simulink model "Force"  (R2016b)
settings: configuration reference "WheelSimConfiguration2016" (kept outside this file)
libraries: dspstat3 x1
settings Model: Creator=At  LastModifiedBy=ateay
settings ConfigSetRef: SourceLocation=Base Workspace

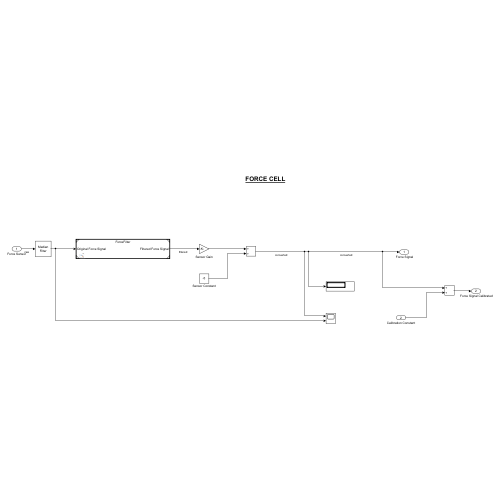
[thumbnail: Simulink's stored preview of the top-level diagram]
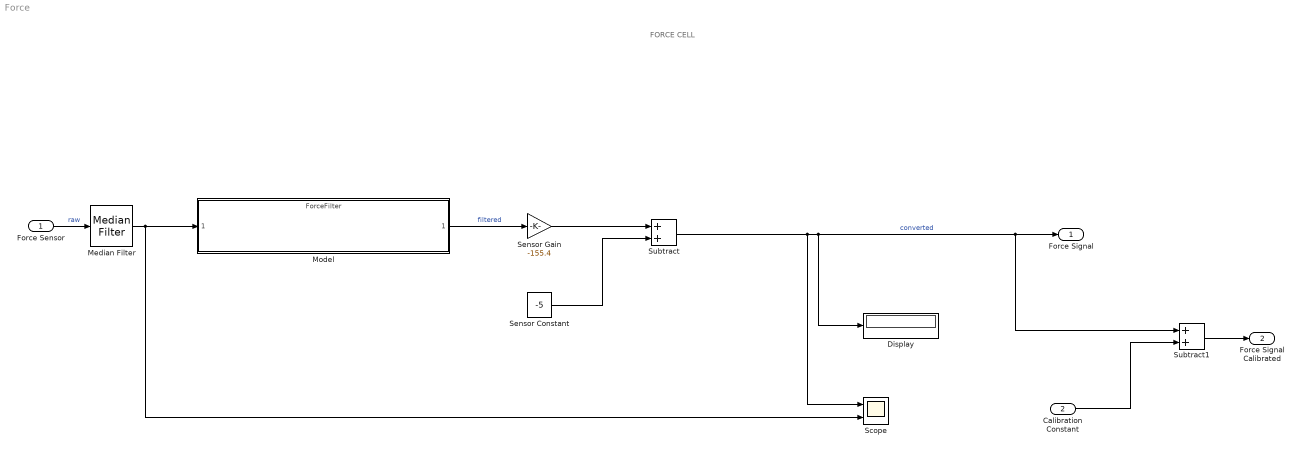
== system Force ==
  note: FORCE CELL
  Force Sensor : Inport
  Calibration Constant : Inport  Port=2
  Display : Display
  Median Filter : dspstat3/Median Filter  WindowLength=3  SimulateUsing=Interpreted execution
  Model : ModelReference  ModelNameDialog=ForceFilter.slx  SimulationMode=Normal  ModelReferenceVersion=1.2
  Scope : Scope  NumInputPorts=2
  Sensor Constant : Constant  Value=-5
  Sensor Gain : Gain  Gain=-155.4
  Subtract : Sum
  Subtract1 : Sum
  " Force Signal" : Outport
  " Force Signal Calibrated" : Outport  Port=2
  wires:
  Force Sensor/1 -> Median Filter/1  "raw"
  Sensor Constant/1 -> Subtract/2
  Sensor Gain/1 -> Subtract/1
  Model/1 -> Sensor Gain/1  "filtered"
  Subtract/1 -> Scope/1, Display/1, Subtract1/1, " Force Signal"/1  "converted"
  Calibration Constant/1 -> Subtract1/2
  Subtract1/1 -> " Force Signal Calibrated"/1
  Median Filter/1 -> Scope/2, Model/1
